simulink model "Rooms_integrated_bus13"  (R2025a)
settings: Solver=VariableStepAuto  StartTime=0.0  StopTime=5  RelTol=1e-3
libraries: spsThreePhaseVIMeasurementLib x53, fl_lib x40, nesl_utility x24, spsThreePhaseSeriesRLCLoadLib x20, spsThreePhasePISectionLineLib x20, spsLoadFlowBusLib x19, simulink x8, spsThreePhaseBreakerLib x8, spspowerguiLib x8, spsThreePhaseTransformerTwoWindingsLib x5, spsThreePhaseSourceLib x5, sps_lib x1
(part 4 of 4)

== system Rooms_integrated_bus13/Power Grid/Bus_9 ==
  Bus : spsThreePhaseVIMeasurementLib/Three-Phase V-I Measurement  VoltageMeasurement=phase-to-phase  SetLabelV=on  LabelV=VB_9  Vpu=off  VpuLL=off  CurrentMeasurement=yes  SetLabelI=on  LabelI=IB_9  Ipu=off  Pbase=100e6  Vbase=500e3  OutputType=Complex  PhasorSimulation=off  PSBequivalent=0
  Bus_ : spsThreePhaseVIMeasurementLib/Three-Phase V-I Measurement  VoltageMeasurement=phase-to-phase  SetLabelV=on  LabelV=V_B9_9  Vpu=off  VpuLL=off  CurrentMeasurement=yes  SetLabelI=on  LabelI=I_B9_9  Ipu=off  Pbase=100e6  Vbase=500e3  OutputType=Complex  PhasorSimulation=off  PSBequivalent=0
  Bus_1 : spsThreePhaseVIMeasurementLib/Three-Phase V-I Measurement  VoltageMeasurement=phase-to-phase  SetLabelV=on  LabelV=V_B9  Vpu=off  VpuLL=off  CurrentMeasurement=yes  SetLabelI=on  LabelI=I_B9  Ipu=off  Pbase=100e6  Vbase=500e3  OutputType=Complex  PhasorSimulation=off  PSBequivalent=0
  Bus_2 : spsThreePhaseVIMeasurementLib/Three-Phase V-I Measurement  VoltageMeasurement=phase-to-phase  SetLabelV=on  LabelV=V_B9__9  Vpu=off  VpuLL=off  CurrentMeasurement=yes  SetLabelI=on  LabelI=I_B9__9  Ipu=off  Pbase=100e6  Vbase=500e3  OutputType=Complex  PhasorSimulation=off  PSBequivalent=0
  Conn1 : PMIOPort  Side=Left
  Conn2 : PMIOPort  Port=2  Side=Right
  Conn3 : PMIOPort  Port=3  Side=Left
  Conn4 : PMIOPort  Port=4  Side=Right
  Conn5 : PMIOPort  Port=5  Side=Right
  Conn6 : PMIOPort  Port=6  Side=Left
  Conn7 : PMIOPort  Port=7  Side=Right
  Conn8 : PMIOPort  Port=8  Side=Right
  Conn9 : PMIOPort  Port=9  Side=Right
  Conn10 : PMIOPort  Port=10  Side=Right
  Conn11 : PMIOPort  Port=11  Side=Right
  Conn12 : PMIOPort  Port=12  Side=Right
  Conn13 : PMIOPort  Port=13  Side=Left
  Conn14 : PMIOPort  Port=14  Side=Left
  Conn15 : PMIOPort  Port=15  Side=Left
  Conn16 : PMIOPort  Port=16  Side=Right
  Conn17 : PMIOPort  Port=17  Side=Right
  Conn18 : PMIOPort  Port=18  Side=Right
  connections:
  Bus/LConn1 -- Conn1/RConn1 -- Conn13/RConn1 -- Bus_/LConn3 -- Bus_1/LConn1 -- Bus_2/LConn3
  Conn3/RConn1 -- Bus/LConn2 -- Bus_/LConn2 -- Conn14/RConn1 -- Bus_1/LConn2 -- Bus_2/LConn2
  Bus_/RConn2 -- Conn8/RConn1
  Bus/RConn2 -- Conn4/RConn1
  Bus/LConn3 -- Conn6/RConn1 -- Bus_/LConn1 -- Conn15/RConn1 -- Bus_1/LConn3 -- Bus_2/LConn1
  Bus/RConn1 -- Conn2/RConn1
  Bus/RConn3 -- Conn5/RConn1
  Conn10/RConn1 -- Bus_1/RConn1
  Conn11/RConn1 -- Bus_1/RConn2
  Conn12/RConn1 -- Bus_1/RConn3
  Conn16/RConn1 -- Bus_2/RConn1
  Conn17/RConn1 -- Bus_2/RConn2
  Conn18/RConn1 -- Bus_2/RConn3
  Conn7/RConn1 -- Bus_/RConn3
  Conn9/RConn1 -- Bus_/RConn1
